simulink model "single_phase_inverter"  (R2020b)
settings: Solver=FixedStepAuto  StartTime=0.0  StopTime=0.3  FixedStep=1e-7  RelTol=1e-3
model workspace (MAT data in the model file):
  ki_u = 1500
  kp_i = 10
  kp_u = 0.1
  m = 0.0001
  n = 1e-06
  time_1 = 0.02
  time_2 = 0.06
undefined symbols (not defined in the file): DiscIntNeverNeededParam
libraries: powerlib x31, pid_lib x6, simulink x2, powerlib_meascontrol x2
settings Model: Creator=csq  LastModifiedBy=csq

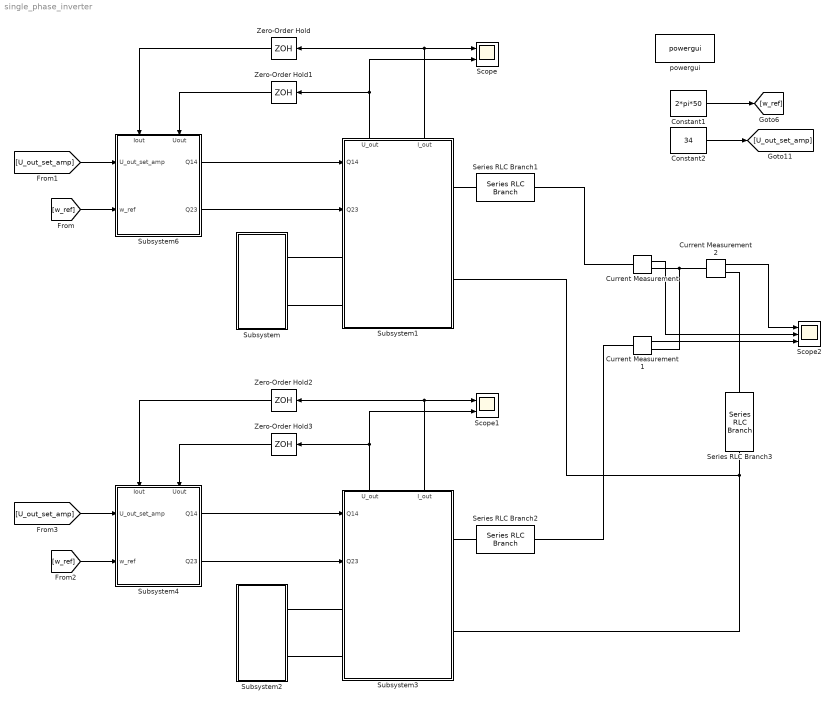
== system single_phase_inverter ==
  Constant1 : Constant  Value=2*pi*50
  Constant2 : Constant  Value=34
  Current Measurement : powerlib/Measurements/Current Measurement  PhasorSimulation=off  OutputType=Complex  PSBequivalent=0
  Current Measurement1 : powerlib/Measurements/Current Measurement  PhasorSimulation=off  OutputType=Complex  PSBequivalent=0
  Current Measurement2 : powerlib/Measurements/Current Measurement  PhasorSimulation=off  OutputType=Complex  PSBequivalent=0
  Scope : Scope  NumInputPorts=2
  Scope1 : Scope  NumInputPorts=2
  Scope2 : Scope  NumInputPorts=3
  Series RLC Branch1 : powerlib/Elements/Series RLC Branch  LConnTagsString=__new0  RConnTagsString=__new0  BranchType=R  Resistance=10e-3  Inductance=1e-3  SetiL0=off  InitialCurrent=0  Capacitance=1e-6  Setx0=off  InitialVoltage=0  Measurements=None
  Series RLC Branch2 : powerlib/Elements/Series RLC Branch  LConnTagsString=__new0  RConnTagsString=__new0  BranchType=R  Resistance=50e-3  Inductance=1e-3  SetiL0=off  InitialCurrent=0  Capacitance=1e-6  Setx0=off  InitialVoltage=0  Measurements=None
  Series RLC Branch3 : powerlib/Elements/Series RLC Branch  LConnTagsString=__new0  RConnTagsString=__new0  BranchType=R  Resistance=12  Inductance=1e-3  SetiL0=off  InitialCurrent=0  Capacitance=1e-6  Setx0=off  InitialVoltage=0  Measurements=None
  Subsystem : Subsystem
  Subsystem1 : Subsystem
      settings: PortSchema="{\"entries\":[{\"content\":{\"sides\":[{\"content\":{\"connectorIds\":[\"In1\",\"In2\",\"LConn1\",\"LConn2\"]},\"type\":\"ConnectorPlacement.EquallySpacedRectSide\",\"uuid\":\"04c4fa80-59b6-45e6-8bac-5e1ed5e22b0f\"},{\"content\":{\"connectorIds\":[\"RConn1\",\"RConn2\"],\"side\":\"RIGHT\"},\"type\":\"ConnectorPlacement.EquallySpacedRectSide\",\"uuid\":\"e41da0a5-fb49-42fc-bfa5-1b3d1422e169\"},{\"content\":{\"connectorIds\":[\"Out1\",\"Out2\"],\"side\":\"TOP\"},\"type\":\"ConnectorPlacement.EquallySpacedRectSide\",\"uuid\":\"69c990dc-7f7f-468a-90c0-dfc1f8754a39\"},{\"content\":{\"connectorIds\":[],\"side\":\"HIDDEN\"},\"type\":\"ConnectorPlacement.EquallySpacedRectSide\",\"uuid\":\"2e87c042-a6fa-4fbf-b837-2a73bea50a04\"}]},\"type\":\"ConnectorPlacement.EquallySpacedConnector\",\"uuid\":\"fc8cbd8d-99a4-408e-86c0-018f445582a3\"}],\"packageUris\":[\"http://schema.mathworks.com/mf0/Connector/R2020b\"],\"version\":\"1.0\"}"
  Subsystem2 : Subsystem
  Subsystem3 : Subsystem
      settings: PortSchema="{\"entries\":[{\"content\":{\"sides\":[{\"content\":{\"connectorIds\":[\"In1\",\"In2\",\"LConn1\",\"LConn2\"]},\"type\":\"ConnectorPlacement.EquallySpacedRectSide\",\"uuid\":\"04c4fa80-59b6-45e6-8bac-5e1ed5e22b0f\"},{\"content\":{\"connectorIds\":[\"RConn1\",\"RConn2\"],\"side\":\"RIGHT\"},\"type\":\"ConnectorPlacement.EquallySpacedRectSide\",\"uuid\":\"e41da0a5-fb49-42fc-bfa5-1b3d1422e169\"},{\"content\":{\"connectorIds\":[\"Out1\",\"Out2\"],\"side\":\"TOP\"},\"type\":\"ConnectorPlacement.EquallySpacedRectSide\",\"uuid\":\"69c990dc-7f7f-468a-90c0-dfc1f8754a39\"},{\"content\":{\"connectorIds\":[],\"side\":\"HIDDEN\"},\"type\":\"ConnectorPlacement.EquallySpacedRectSide\",\"uuid\":\"2e87c042-a6fa-4fbf-b837-2a73bea50a04\"}]},\"type\":\"ConnectorPlacement.EquallySpacedConnector\",\"uuid\":\"fc8cbd8d-99a4-408e-86c0-018f445582a3\"}],\"packageUris\":[\"http://schema.mathworks.com/mf0/Connector/R2020b\"],\"version\":\"1.0\"}"
  Subsystem4 : Subsystem
      settings: PortSchema="{\"entries\":[{\"content\":{\"sides\":[{\"content\":{\"connectorIds\":[\"In1\",\"In2\"]},\"type\":\"ConnectorPlacement.EquallySpacedRectSide\",\"uuid\":\"624b767b-a834-4e37-aaa6-33de15262b98\"},{\"content\":{\"connectorIds\":[\"Out1\",\"Out2\"],\"side\":\"RIGHT\"},\"type\":\"ConnectorPlacement.EquallySpacedRectSide\",\"uuid\":\"636cd8d4-39b1-4a76-b8fe-b877b788af90\"},{\"content\":{\"connectorIds\":[\"In3\",\"In4\"],\"side\":\"TOP\"},\"type\":\"ConnectorPlacement.EquallySpacedRectSide\",\"uuid\":\"27128ec8-804f-46a4-a20c-7bc453791419\"},{\"content\":{\"connectorIds\":[],\"side\":\"HIDDEN\"},\"type\":\"ConnectorPlacement.EquallySpacedRectSide\",\"uuid\":\"cec971ba-b3f6-4dcf-9360-3ebb47930643\"}]},\"type\":\"ConnectorPlacement.EquallySpacedConnector\",\"uuid\":\"76619d1a-6bef-4a4f-ace2-d43c42a45d1f\"}],\"packageUris\":[\"http://schema.mathworks.com/mf0/Connector/R2020b\"],\"version\":\"1.0\"}"
  Subsystem6 : Subsystem
      settings: PortSchema="{\"entries\":[{\"content\":{\"sides\":[{\"content\":{\"connectorIds\":[\"In1\",\"In2\"]},\"type\":\"ConnectorPlacement.EquallySpacedRectSide\",\"uuid\":\"624b767b-a834-4e37-aaa6-33de15262b98\"},{\"content\":{\"connectorIds\":[\"Out1\",\"Out2\"],\"side\":\"RIGHT\"},\"type\":\"ConnectorPlacement.EquallySpacedRectSide\",\"uuid\":\"636cd8d4-39b1-4a76-b8fe-b877b788af90\"},{\"content\":{\"connectorIds\":[\"In3\",\"In4\"],\"side\":\"TOP\"},\"type\":\"ConnectorPlacement.EquallySpacedRectSide\",\"uuid\":\"27128ec8-804f-46a4-a20c-7bc453791419\"},{\"content\":{\"connectorIds\":[],\"side\":\"HIDDEN\"},\"type\":\"ConnectorPlacement.EquallySpacedRectSide\",\"uuid\":\"cec971ba-b3f6-4dcf-9360-3ebb47930643\"}]},\"type\":\"ConnectorPlacement.EquallySpacedConnector\",\"uuid\":\"76619d1a-6bef-4a4f-ace2-d43c42a45d1f\"}],\"packageUris\":[\"http://schema.mathworks.com/mf0/Connector/R2020b\"],\"version\":\"1.0\"}"
  Zero-Order Hold{,1..3} (4 alike) : ZeroOrderHold  SampleTime=1/20e3
  powergui : powerlib/powergui  Priority=1  SimulationMode=Discrete  SampleTime=1e-7  frequency=60  Iterations=50  frequencyindice=0  Pbase=100e6  ErrMax=1e-4  UnitsV=kV  UnitsW=MW  buscounter=0  FunctionMessages=off  echomessages=off  EnableUseOfTLC=off  CurrentSourceSwitches=off  DisableSnubberDevices=off  DisableRonSwitches=off  DisableVfSwitches=off  DisplayEquations=off  AutomaticDiscreteSolvers=off  SolverType=Tustin/Backward Euler (TBE)  Interpol=off  ExternalGateDelay=off  methode=off  Ts=100  x0status=blocks  SPID=on  SwTol=0  HookPort=off  NonlinearTolerance=1e-4  nMaxIteration=100  ContinueOnMaxIteration=off  RestoreLinks=warning  ResistiveCurrentMeasurement=off  Frange=[0:2:500]  Ylog=off  Xlog=on  ShowGrid=off  save=off  variable=ZData  structure=0  ZoomFFT=off  StartTime=0.0  cycles=1  DisplayStyle=1  fundamental=60  FreqAxis=off  MaxFrequency=1000  frequencyindicesteady=1  RmsSteady=1  display=off
  wires:
  Constant1/1 -> [w_ref]
  Constant2/1 -> [U_out_set_amp]
  [w_ref] -> Subsystem6/2(w_ref)
  [U_out_set_amp] -> Subsystem6/1(U_out_set_amp)
  Subsystem6/1(Q14) -> Subsystem1/1(Q14)
  Subsystem6/2(Q23) -> Subsystem1/2(Q23)
  Subsystem1/1(U_out) -> Scope/2, Zero-Order Hold1/1
  Subsystem1/2(I_out) -> Scope/1, Zero-Order Hold/1
  Zero-Order Hold1/1 -> Subsystem6/4(Uout)
  Zero-Order Hold/1 -> Subsystem6/3(Iout)
  Zero-Order Hold2/1 -> Subsystem4/3(Iout)
  Zero-Order Hold3/1 -> Subsystem4/4(Uout)
  Subsystem3/2(I_out) -> Zero-Order Hold2/1, Scope1/1
  Subsystem3/1(U_out) -> Zero-Order Hold3/1, Scope1/2
  [U_out_set_amp] -> Subsystem4/1(U_out_set_amp)
  [w_ref] -> Subsystem4/2(w_ref)
  Subsystem4/1(Q14) -> Subsystem3/1(Q14)
  Subsystem4/2(Q23) -> Subsystem3/2(Q23)
  Current Measurement2/1 -> Scope2/1
  Current Measurement/1 -> Scope2/2
  Current Measurement1/1 -> Scope2/3
  connections:
  Subsystem/RConn1 -- Subsystem1/LConn1
  Subsystem/RConn2 -- Subsystem1/LConn2
  Subsystem2/RConn2 -- Subsystem3/LConn2
  Subsystem2/RConn1 -- Subsystem3/LConn1
  Subsystem1/RConn2 -- Series RLC Branch3/LConn1 -- Subsystem3/RConn2
  Current Measurement/RConn1 -- Current Measurement1/RConn1 -- Current Measurement2/LConn1
  Series RLC Branch3/RConn1 -- Current Measurement2/RConn1
  Subsystem1/RConn1 -- Series RLC Branch1/RConn1
  Subsystem3/RConn1 -- Series RLC Branch2/RConn1
  Series RLC Branch1/LConn1 -- Current Measurement/LConn1
  Series RLC Branch2/LConn1 -- Current Measurement1/LConn1

== system single_phase_inverter/Subsystem ==
  DC Voltage Source1 : powerlib/Electrical Sources/DC Voltage Source  Amplitude=48  Measurements=None
  Series RLC Branch2 : powerlib/Elements/Series RLC Branch  LConnTagsString=__new0  RConnTagsString=__new0  BranchType=R  Resistance=5e-3  Inductance=1e-3  SetiL0=off  InitialCurrent=0  Capacitance=220e-6  Setx0=off  InitialVoltage=0  Measurements=None
  Series RLC Branch6 : powerlib/Elements/Series RLC Branch  LConnTagsString=__new0  RConnTagsString=__new0  BranchType=RC  Resistance=5e-3  Inductance=1e-3  SetiL0=off  InitialCurrent=0  Capacitance=220e-6  Setx0=off  InitialVoltage=0  Measurements=None
  DC+ : PMIOPort  Side=Right
  DC- : PMIOPort  Port=2  Side=Right
  connections:
  DC Voltage Source1/RConn1 -- Series RLC Branch2/RConn1
  DC Voltage Source1/LConn1 -- Series RLC Branch6/RConn1 -- DC-/RConn1
  Series RLC Branch6/LConn1 -- Series RLC Branch2/LConn1 -- DC+/RConn1

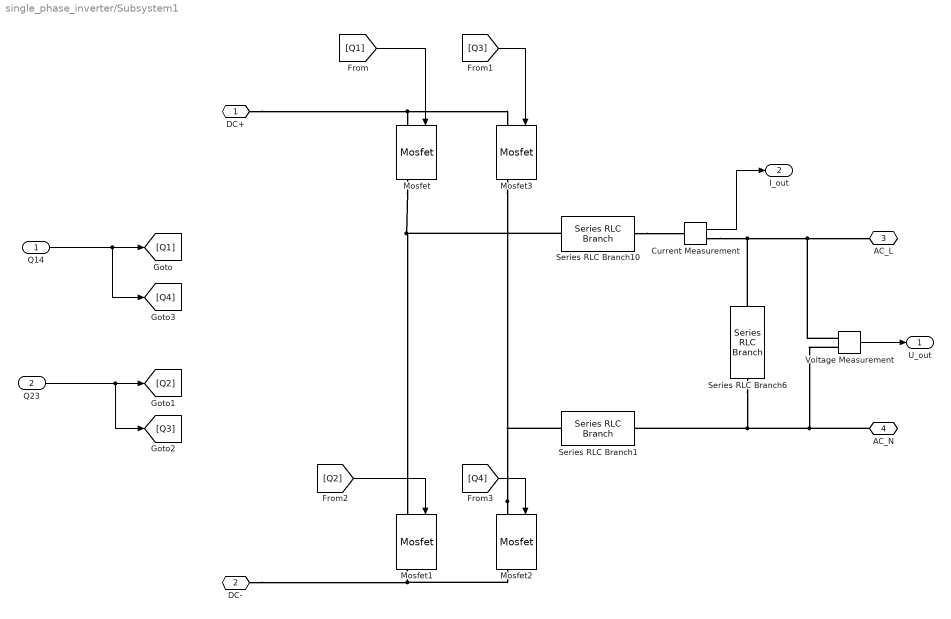
== system single_phase_inverter/Subsystem1 ==
  Q14 : Inport
  Q23 : Inport  Port=2
  Current Measurement : powerlib/Measurements/Current Measurement  PhasorSimulation=off  OutputType=Complex  PSBequivalent=0
  Mosfet{,1..3} (4 alike) : powerlib/Power Electronics/Mosfet  Ron=0.1  Lon=0  Rd=0.01  Vfd=0  IC=0  Rs=1e5  Cs=inf  Measurements=on
  Series RLC Branch1 : powerlib/Elements/Series RLC Branch  LConnTagsString=__new0  RConnTagsString=__new0  BranchType=RL  Resistance=10e-3  Inductance=1e-3  SetiL0=off  InitialCurrent=0  Capacitance=1e-6  Setx0=off  InitialVoltage=0  Measurements=None
  Series RLC Branch10 : powerlib/Elements/Series RLC Branch  LConnTagsString=__new0  RConnTagsString=__new0  BranchType=RL  Resistance=10e-3  Inductance=1e-3  SetiL0=off  InitialCurrent=0  Capacitance=1e-6  Setx0=off  InitialVoltage=0  Measurements=None
  Series RLC Branch6 : powerlib/Elements/Series RLC Branch  LConnTagsString=__new0  RConnTagsString=__new0  BranchType=RC  Resistance=5e-3  Inductance=1e-3  SetiL0=off  InitialCurrent=0  Capacitance=2e-6  Setx0=off  InitialVoltage=0  Measurements=None
  Voltage Measurement : powerlib/Measurements/Voltage Measurement  PhasorSimulation=off  OutputType=Complex  PSBequivalent=0
  DC+ : PMIOPort  Side=Left
  DC- : PMIOPort  Port=2  Side=Left
  AC_L : PMIOPort  Port=3  Side=Right
  AC_N : PMIOPort  Port=4  Side=Right
  U_out : Outport
  I_out : Outport  Port=2
  wires:
  Current Measurement/1 -> I_out/1
  Voltage Measurement/1 -> U_out/1
  [Q1] -> Mosfet/1
  [Q3] -> Mosfet3/1
  [Q2] -> Mosfet1/1
  [Q4] -> Mosfet2/1
  Q23/1 -> [Q3], [Q2]
  Q14/1 -> [Q4], [Q1]
  connections:
  DC-/RConn1 -- Mosfet1/RConn1 -- Mosfet2/RConn1
  DC+/RConn1 -- Mosfet/LConn1 -- Mosfet3/LConn1
  Series RLC Branch6/LConn1 -- Voltage Measurement/LConn1 -- AC_L/RConn1 -- Current Measurement/RConn1
  Mosfet2/LConn1 -- Mosfet3/RConn1 -- Series RLC Branch1/LConn1
  Series RLC Branch10/LConn1 -- Mosfet1/LConn1 -- Mosfet/RConn1
  AC_N/RConn1 -- Series RLC Branch6/RConn1 -- Series RLC Branch1/RConn1 -- Voltage Measurement/LConn2
  Series RLC Branch10/RConn1 -- Current Measurement/LConn1

== system single_phase_inverter/Subsystem2 ==
  DC Voltage Source1 : powerlib/Electrical Sources/DC Voltage Source  Amplitude=48  Measurements=None
  Series RLC Branch2 : powerlib/Elements/Series RLC Branch  LConnTagsString=__new0  RConnTagsString=__new0  BranchType=R  Resistance=5e-3  Inductance=1e-3  SetiL0=off  InitialCurrent=0  Capacitance=220e-6  Setx0=off  InitialVoltage=0  Measurements=None
  Series RLC Branch6 : powerlib/Elements/Series RLC Branch  LConnTagsString=__new0  RConnTagsString=__new0  BranchType=RC  Resistance=5e-3  Inductance=1e-3  SetiL0=off  InitialCurrent=0  Capacitance=220e-6  Setx0=off  InitialVoltage=0  Measurements=None
  DC+ : PMIOPort  Side=Right
  DC- : PMIOPort  Port=2  Side=Right
  connections:
  DC+/RConn1 -- Series RLC Branch6/LConn1 -- Series RLC Branch2/LConn1
  DC-/RConn1 -- Series RLC Branch6/RConn1 -- DC Voltage Source1/LConn1
  DC Voltage Source1/RConn1 -- Series RLC Branch2/RConn1

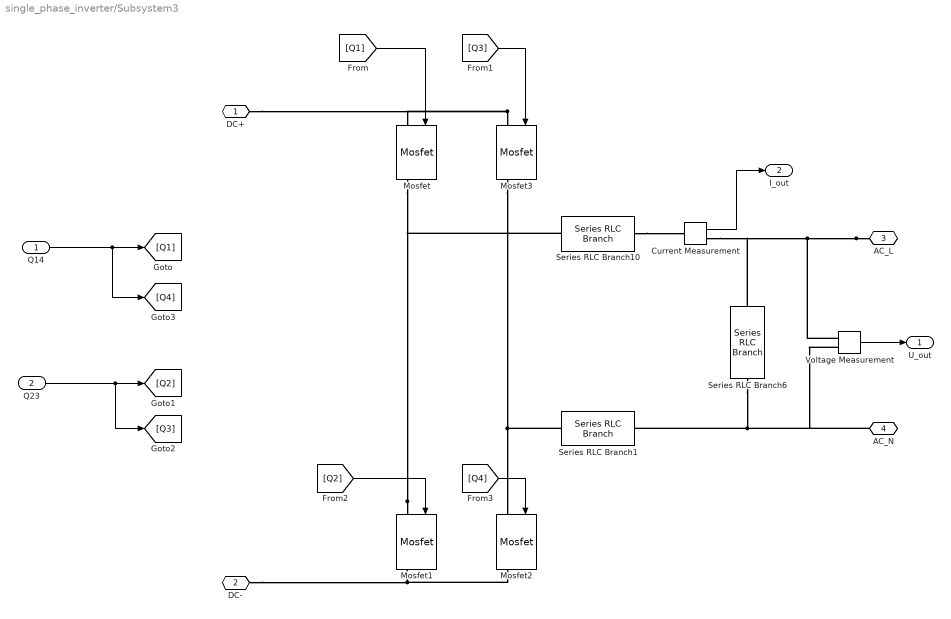
== system single_phase_inverter/Subsystem3 ==
  Q14 : Inport
  Q23 : Inport  Port=2
  Current Measurement : powerlib/Measurements/Current Measurement  PhasorSimulation=off  OutputType=Complex  PSBequivalent=0
  Mosfet{,1..3} (4 alike) : powerlib/Power Electronics/Mosfet  Ron=0.1  Lon=0  Rd=0.01  Vfd=0  IC=0  Rs=1e5  Cs=inf  Measurements=on
  Series RLC Branch1 : powerlib/Elements/Series RLC Branch  LConnTagsString=__new0  RConnTagsString=__new0  BranchType=RL  Resistance=10e-3  Inductance=1e-3  SetiL0=off  InitialCurrent=0  Capacitance=1e-6  Setx0=off  InitialVoltage=0  Measurements=None
  Series RLC Branch10 : powerlib/Elements/Series RLC Branch  LConnTagsString=__new0  RConnTagsString=__new0  BranchType=RL  Resistance=10e-3  Inductance=1e-3  SetiL0=off  InitialCurrent=0  Capacitance=1e-6  Setx0=off  InitialVoltage=0  Measurements=None
  Series RLC Branch6 : powerlib/Elements/Series RLC Branch  LConnTagsString=__new0  RConnTagsString=__new0  BranchType=RC  Resistance=5e-3  Inductance=1e-3  SetiL0=off  InitialCurrent=0  Capacitance=2e-6  Setx0=off  InitialVoltage=0  Measurements=None
  Voltage Measurement : powerlib/Measurements/Voltage Measurement  PhasorSimulation=off  OutputType=Complex  PSBequivalent=0
  DC+ : PMIOPort  Side=Left
  DC- : PMIOPort  Port=2  Side=Left
  AC_L : PMIOPort  Port=3  Side=Right
  AC_N : PMIOPort  Port=4  Side=Right
  U_out : Outport
  I_out : Outport  Port=2
  wires:
  Q14/1 -> [Q1], [Q4]
  Q23/1 -> [Q2], [Q3]
  [Q4] -> Mosfet2/1
  [Q2] -> Mosfet1/1
  [Q3] -> Mosfet3/1
  [Q1] -> Mosfet/1
  Voltage Measurement/1 -> U_out/1
  Current Measurement/1 -> I_out/1
  connections:
  Series RLC Branch10/RConn1 -- Current Measurement/LConn1
  Voltage Measurement/LConn2 -- AC_N/RConn1 -- Series RLC Branch1/RConn1 -- Series RLC Branch6/RConn1
  Mosfet1/LConn1 -- Mosfet/RConn1 -- Series RLC Branch10/LConn1
  Series RLC Branch1/LConn1 -- Mosfet2/LConn1 -- Mosfet3/RConn1
  AC_L/RConn1 -- Voltage Measurement/LConn1 -- Current Measurement/RConn1 -- Series RLC Branch6/LConn1
  Mosfet3/LConn1 -- Mosfet/LConn1 -- DC+/RConn1
  Mosfet2/RConn1 -- Mosfet1/RConn1 -- DC-/RConn1

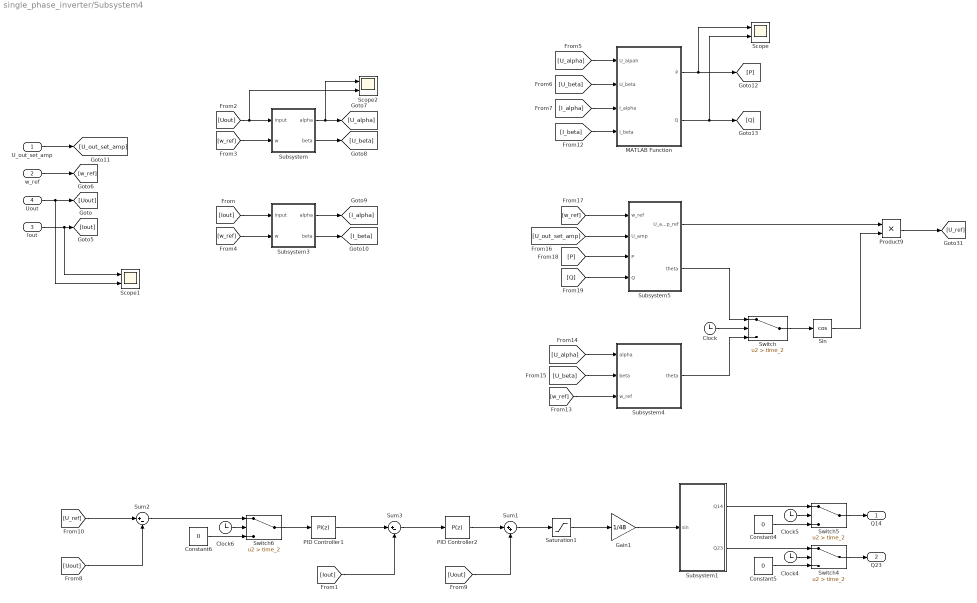
== system single_phase_inverter/Subsystem4 ==
  U_out_set_amp : Inport
  w_ref : Inport  Port=2
  Iout : Inport  Port=3
  Uout : Inport  Port=4
  Clock{,4..6} (4 alike) : Clock
  Constant4 : Constant  Value=0
  Constant5 : Constant  Value=0
  Constant6 : Constant  Value=0
  Gain1 : Gain  Gain=1/48
  MATLAB Function : MATLAB Function  TreatAsAtomicUnit=on
  PID Controller1 : pid_lib/PID Controller  Controller=PI  Form=Parallel  TimeDomain=Discrete-time  UseExternalTs=off  SampleTime=1/20e3  IntegratorMethod=Forward Euler  FilterMethod=Forward Euler  ControllerParametersSource=internal  P=kp_u  I=ki_u  D=0  UseFilter=on  N=100  TunerSelectOption=Transfer Function Based (PID Tuner App)  InitialConditionSource=internal  InitialConditionForIntegrator=0  InitialConditionForFilter=0  DifferentiatorICPrevScaledInput=0  ExternalReset=none  TrackingMode=off  Kt=1  LimitOutput=on  SatLimitsSource=internal  UpperSaturationLimit=50  LowerSaturationLimit=-50  LinearizeAsGain=on  AntiWindupMode=none  Kb=1  POutMin=[]  POutMax=[]  IOutMin=[]  IOutMax=[]  DOutMin=[]  DOutMax=[]  NOutMin=[]  NOutMax=[]  SumOutMin=[]  SumOutMax=[]  SaturationOutMin=[]  SaturationOutMax=[]  PParamMin=[]  PParamMax=[]  IParamMin=[]  IParamMax=[]  DParamMin=[]  DParamMax=[]  NParamMin=[]  NParamMax=[]  KbParamMin=[]  KbParamMax=[]  KtParamMin=[]  KtParamMax=[]  KbOutMin=[]  KbOutMax=[]  KtOutMin=[]  KtOutMax=[]  IntegratorOutMin=[]  IntegratorOutMax=[]  FilterOutMin=[]  FilterOutMax=[]  SumI1OutMin=[]  SumI1OutMax=[]  SumI2OutMin=[]  SumI2OutMax=[]  SumI3OutMin=[]  SumI3OutMax=[]  SumI4OutMin=[]  SumI4OutMax=[]  SumDOutMin=[]  SumDOutMax=[]  DifferentiatorOutMin=[]  DifferentiatorOutMax=[]  FilterDiffOutCoefMin=[]  FilterDiffOutCoefMax=[]  ReciprocalOutMin=[]  ReciprocalOutMax=[]  SumDenOutMin=[]  SumDenOutMax=[]  SumNumOutMin=[]  SumNumOutMax=[]  DivideOutMin=[]  DivideOutMax=[]  UdiffTsProdOutMin=[]  UdiffTsProdOutMax=[]  NTsProdOutMin=[]  NTsProdOutMax=[]  UintegralTsProdOutMin=[]  UintegralTsProdOutMax=[]  UngainTsProdOutMin=[]  UngainTsProdOutMax=[]  IntegratorContinuousStateAttributes=''  IntegratorStateMustResolveToSignalObject=off  IntegratorRTWStateStorageClass=Auto  FilterContinuousStateAttributes=''  FilterStateMustResolveToSignalObject=off  FilterRTWStateStorageClass=Auto  ParallelPVariant=InternalParameters  IdealPVariant=Disabled  IVariant=InternalParameters  DVariant=Disabled  IntegratorVariant=Discrete  SatVariant=Enabled  AWVariant=Passthrough  PCopyVariant=Disabled  TRVariant=Disabled  FdbkBlocksVariant=Forward  IdealPFdbkVariant=Disabled  SatFdbkVariant=Disabled  DerivativeFilterVariant=Disabled  NVariant=Disabled  NCopyVariant=Disabled_SignalSpec  FilterICVariant=Disabled  IntegratorICVariant=InternalICs  ExternalResetVariant=Disabled  TRSumVariant=Passthrough  SumFdbkVariant=Disabled  SumVariant=Sum_PI  TsampFilterVariant=InternalTs  TsampNgainVariant=Passthrough  TsampIntegralVariant=Passthrough  ExternalSaturationOutDataTypeStr=Inherit: Same as second input
  PID Controller2 : pid_lib/PID Controller  Controller=P  Form=Parallel  TimeDomain=Discrete-time  UseExternalTs=off  SampleTime=1/20e3  IntegratorMethod=Forward Euler  FilterMethod=Forward Euler  ControllerParametersSource=internal  P=kp_i  I=10  D=0  UseFilter=on  N=100  TunerSelectOption=Transfer Function Based (PID Tuner App)  InitialConditionSource=internal  InitialConditionForIntegrator=0  InitialConditionForFilter=0  DifferentiatorICPrevScaledInput=0  ExternalReset=none  TrackingMode=off  Kt=1  LimitOutput=off  SatLimitsSource=internal  UpperSaturationLimit=inf  LowerSaturationLimit=-inf  LinearizeAsGain=on  AntiWindupMode=none  Kb=1  POutMin=[]  POutMax=[]  IOutMin=[]  IOutMax=[]  DOutMin=[]  DOutMax=[]  NOutMin=[]  NOutMax=[]  SumOutMin=[]  SumOutMax=[]  SaturationOutMin=[]  SaturationOutMax=[]  PParamMin=[]  PParamMax=[]  IParamMin=[]  IParamMax=[]  DParamMin=[]  DParamMax=[]  NParamMin=[]  NParamMax=[]  KbParamMin=[]  KbParamMax=[]  KtParamMin=[]  KtParamMax=[]  KbOutMin=[]  KbOutMax=[]  KtOutMin=[]  KtOutMax=[]  IntegratorOutMin=[]  IntegratorOutMax=[]  FilterOutMin=[]  FilterOutMax=[]  SumI1OutMin=[]  SumI1OutMax=[]  SumI2OutMin=[]  SumI2OutMax=[]  SumI3OutMin=[]  SumI3OutMax=[]  SumI4OutMin=[]  SumI4OutMax=[]  SumDOutMin=[]  SumDOutMax=[]  DifferentiatorOutMin=[]  DifferentiatorOutMax=[]  FilterDiffOutCoefMin=[]  FilterDiffOutCoefMax=[]  ReciprocalOutMin=[]  ReciprocalOutMax=[]  SumDenOutMin=[]  SumDenOutMax=[]  SumNumOutMin=[]  SumNumOutMax=[]  DivideOutMin=[]  DivideOutMax=[]  UdiffTsProdOutMin=[]  UdiffTsProdOutMax=[]  NTsProdOutMin=[]  NTsProdOutMax=[]  UintegralTsProdOutMin=[]  UintegralTsProdOutMax=[]  UngainTsProdOutMin=[]  UngainTsProdOutMax=[]  IntegratorContinuousStateAttributes=''  IntegratorStateMustResolveToSignalObject=off  IntegratorRTWStateStorageClass=Auto  FilterContinuousStateAttributes=''  FilterStateMustResolveToSignalObject=off  FilterRTWStateStorageClass=Auto  ParallelPVariant=InternalParameters  IdealPVariant=Disabled  IVariant=Disabled  DVariant=Disabled  IntegratorVariant=Disabled  SatVariant=Disabled  AWVariant=Disabled  PCopyVariant=Disabled  TRVariant=Disabled  FdbkBlocksVariant=Forward  IdealPFdbkVariant=Disabled  SatFdbkVariant=Disabled  DerivativeFilterVariant=Disabled  NVariant=Disabled  NCopyVariant=Disabled_SignalSpec  FilterICVariant=Disabled  IntegratorICVariant=Disabled  ExternalResetVariant=Disabled  TRSumVariant=Passthrough  SumFdbkVariant=Disabled  SumVariant=Passthrough_P  TsampFilterVariant=InternalTs  TsampNgainVariant=Passthrough  TsampIntegralVariant=Disabled_SignalSpec  ExternalSaturationOutDataTypeStr=Inherit: Same as second input
  Product9 : Product
  Saturation1 : Saturate  UpperLimit=48  LowerLimit=-48
  Scope : Scope  NumInputPorts=2
  Scope1 : Scope  NumInputPorts=2
  Scope2 : Scope  NumInputPorts=2
  Sin : Trigonometry  Operator=cos
  Subsystem : Subsystem
  Subsystem1 : Subsystem
  Subsystem3 : Subsystem
  Subsystem4 : Subsystem
  Subsystem5 : Subsystem
  Sum1 : Sum  Inputs=|++
  Sum2 : Sum  Inputs=|+-
  Sum3 : Sum  Inputs=|+-
  Switch{,4..6} (4 alike) : Switch  Criteria=u2 > Threshold  Threshold=time_2
  Q14 : Outport
  Q23 : Outport  Port=2
  wires:
  [U_out_set_amp] -> Subsystem5/2(U_amp)
  U_out_set_amp/1 -> [U_out_set_amp]
  w_ref/1 -> [w_ref]
  Uout/1 -> [Uout], Scope1/2
  Iout/1 -> [Iout], Scope1/1
  [U_alpha] -> Subsystem4/1(alpha)
  [U_beta] -> Subsystem4/2(beta)
  Product9/1 -> [U_ref]
  [w_ref] -> Subsystem4/3(w_ref)
  Subsystem3/2(beta) -> [I_beta]
  Subsystem/1(alpha) -> [U_alpha], Scope2/1
  [w_ref] -> Subsystem5/1(w_ref)
  [Q] -> Subsystem5/4(Q)
  [U_alpha] -> MATLAB Function/1(U_alpah)
  Subsystem5/2(theta) -> Switch/1
  Subsystem3/1(alpha) -> [I_alpha]
  [U_beta] -> MATLAB Function/2(U_beta)
  Clock/1 -> Switch/2
  [I_alpha] -> MATLAB Function/3(I_alpha)
  [Iout] -> Subsystem3/1(input)
  [P] -> Subsystem5/3(P)
  [w_ref] -> Subsystem3/2(w)
  Subsystem5/1(U_amp_ref) -> Product9/1
  Subsystem4/1(theta) -> Switch/3
  [Uout] -> Subsystem/1(input), Scope2/2
  Switch/1 -> Sin/1
  Sin/1 -> Product9/2
  Subsystem/2(beta) -> [U_beta]
  MATLAB Function/1(P) -> [P], Scope/1
  MATLAB Function/2(Q) -> [Q], Scope/2
  [I_beta] -> MATLAB Function/4(I_beta)
  [w_ref] -> Subsystem/2(w)
  Constant6/1 -> Switch6/3
  Gain1/1 -> Subsystem1/1(sin)
  Constant4/1 -> Switch5/3
  [Uout] -> Sum1/2
  Switch4/1 -> Q23/1
  Subsystem1/1(Q14) -> Switch5/1
  Switch6/1 -> PID Controller1/1
  Sum2/1 -> Switch6/1
  Subsystem1/2(Q23) -> Switch4/1
  PID Controller2/1 -> Sum1/1
  Clock4/1 -> Switch4/2
  Switch5/1 -> Q14/1
  Constant5/1 -> Switch4/3
  [U_ref] -> Sum2/1
  PID Controller1/1 -> Sum3/1
  Clock6/1 -> Switch6/2
  Saturation1/1 -> Gain1/1
  [Iout] -> Sum3/2
  Clock5/1 -> Switch5/2
  Sum3/1 -> PID Controller2/1
  Sum1/1 -> Saturation1/1
  [Uout] -> Sum2/2

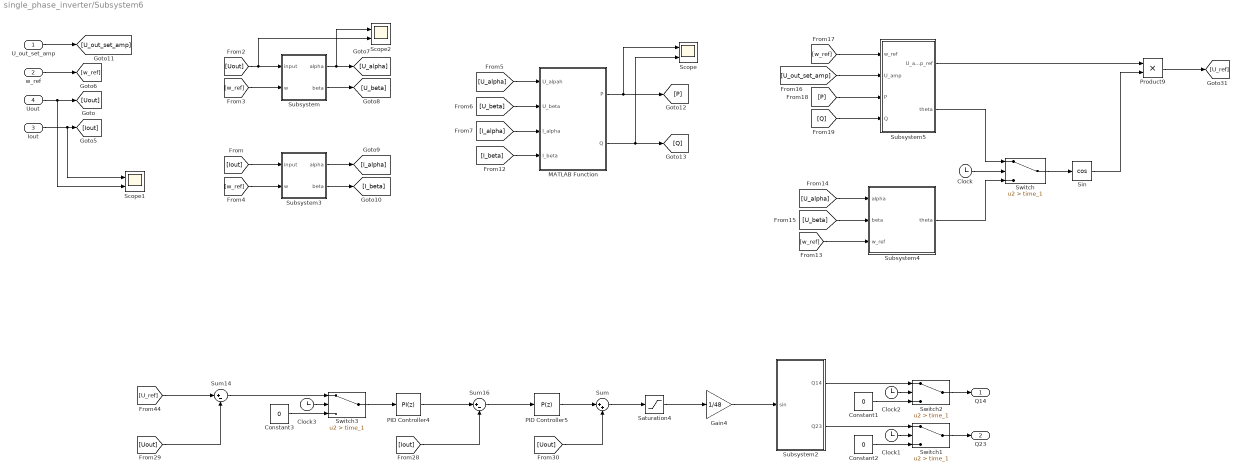
== system single_phase_inverter/Subsystem6 ==
  U_out_set_amp : Inport
  w_ref : Inport  Port=2
  Iout : Inport  Port=3
  Uout : Inport  Port=4
  Clock{,1..3} (4 alike) : Clock
  Constant1 : Constant  Value=0
  Constant2 : Constant  Value=0
  Constant3 : Constant  Value=0
  Gain4 : Gain  Gain=1/48
  MATLAB Function : MATLAB Function  TreatAsAtomicUnit=on
  PID Controller4 : pid_lib/PID Controller  Controller=PI  Form=Parallel  TimeDomain=Discrete-time  UseExternalTs=off  SampleTime=1/20e3  IntegratorMethod=Forward Euler  FilterMethod=Forward Euler  ControllerParametersSource=internal  P=kp_u  I=ki_u  D=0  UseFilter=on  N=100  TunerSelectOption=Transfer Function Based (PID Tuner App)  InitialConditionSource=internal  InitialConditionForIntegrator=0  InitialConditionForFilter=0  DifferentiatorICPrevScaledInput=0  ExternalReset=none  TrackingMode=off  Kt=1  LimitOutput=on  SatLimitsSource=internal  UpperSaturationLimit=50  LowerSaturationLimit=-50  LinearizeAsGain=on  AntiWindupMode=none  Kb=1  POutMin=[]  POutMax=[]  IOutMin=[]  IOutMax=[]  DOutMin=[]  DOutMax=[]  NOutMin=[]  NOutMax=[]  SumOutMin=[]  SumOutMax=[]  SaturationOutMin=[]  SaturationOutMax=[]  PParamMin=[]  PParamMax=[]  IParamMin=[]  IParamMax=[]  DParamMin=[]  DParamMax=[]  NParamMin=[]  NParamMax=[]  KbParamMin=[]  KbParamMax=[]  KtParamMin=[]  KtParamMax=[]  KbOutMin=[]  KbOutMax=[]  KtOutMin=[]  KtOutMax=[]  IntegratorOutMin=[]  IntegratorOutMax=[]  FilterOutMin=[]  FilterOutMax=[]  SumI1OutMin=[]  SumI1OutMax=[]  SumI2OutMin=[]  SumI2OutMax=[]  SumI3OutMin=[]  SumI3OutMax=[]  SumI4OutMin=[]  SumI4OutMax=[]  SumDOutMin=[]  SumDOutMax=[]  DifferentiatorOutMin=[]  DifferentiatorOutMax=[]  FilterDiffOutCoefMin=[]  FilterDiffOutCoefMax=[]  ReciprocalOutMin=[]  ReciprocalOutMax=[]  SumDenOutMin=[]  SumDenOutMax=[]  SumNumOutMin=[]  SumNumOutMax=[]  DivideOutMin=[]  DivideOutMax=[]  UdiffTsProdOutMin=[]  UdiffTsProdOutMax=[]  NTsProdOutMin=[]  NTsProdOutMax=[]  UintegralTsProdOutMin=[]  UintegralTsProdOutMax=[]  UngainTsProdOutMin=[]  UngainTsProdOutMax=[]  IntegratorContinuousStateAttributes=''  IntegratorStateMustResolveToSignalObject=off  IntegratorRTWStateStorageClass=Auto  FilterContinuousStateAttributes=''  FilterStateMustResolveToSignalObject=off  FilterRTWStateStorageClass=Auto  ParallelPVariant=InternalParameters  IdealPVariant=Disabled  IVariant=InternalParameters  DVariant=Disabled  IntegratorVariant=Discrete  SatVariant=Enabled  AWVariant=Passthrough  PCopyVariant=Disabled  TRVariant=Disabled  FdbkBlocksVariant=Forward  IdealPFdbkVariant=Disabled  SatFdbkVariant=Disabled  DerivativeFilterVariant=Disabled  NVariant=Disabled  NCopyVariant=Disabled_SignalSpec  FilterICVariant=Disabled  IntegratorICVariant=InternalICs  ExternalResetVariant=Disabled  TRSumVariant=Passthrough  SumFdbkVariant=Disabled  SumVariant=Sum_PI  TsampFilterVariant=InternalTs  TsampNgainVariant=Passthrough  TsampIntegralVariant=Passthrough  ExternalSaturationOutDataTypeStr=Inherit: Same as second input
  PID Controller5 : pid_lib/PID Controller  Controller=P  Form=Parallel  TimeDomain=Discrete-time  UseExternalTs=off  SampleTime=1/20e3  IntegratorMethod=Forward Euler  FilterMethod=Forward Euler  ControllerParametersSource=internal  P=kp_i  I=10  D=0  UseFilter=on  N=100  TunerSelectOption=Transfer Function Based (PID Tuner App)  InitialConditionSource=internal  InitialConditionForIntegrator=0  InitialConditionForFilter=0  DifferentiatorICPrevScaledInput=0  ExternalReset=none  TrackingMode=off  Kt=1  LimitOutput=off  SatLimitsSource=internal  UpperSaturationLimit=inf  LowerSaturationLimit=-inf  LinearizeAsGain=on  AntiWindupMode=none  Kb=1  POutMin=[]  POutMax=[]  IOutMin=[]  IOutMax=[]  DOutMin=[]  DOutMax=[]  NOutMin=[]  NOutMax=[]  SumOutMin=[]  SumOutMax=[]  SaturationOutMin=[]  SaturationOutMax=[]  PParamMin=[]  PParamMax=[]  IParamMin=[]  IParamMax=[]  DParamMin=[]  DParamMax=[]  NParamMin=[]  NParamMax=[]  KbParamMin=[]  KbParamMax=[]  KtParamMin=[]  KtParamMax=[]  KbOutMin=[]  KbOutMax=[]  KtOutMin=[]  KtOutMax=[]  IntegratorOutMin=[]  IntegratorOutMax=[]  FilterOutMin=[]  FilterOutMax=[]  SumI1OutMin=[]  SumI1OutMax=[]  SumI2OutMin=[]  SumI2OutMax=[]  SumI3OutMin=[]  SumI3OutMax=[]  SumI4OutMin=[]  SumI4OutMax=[]  SumDOutMin=[]  SumDOutMax=[]  DifferentiatorOutMin=[]  DifferentiatorOutMax=[]  FilterDiffOutCoefMin=[]  FilterDiffOutCoefMax=[]  ReciprocalOutMin=[]  ReciprocalOutMax=[]  SumDenOutMin=[]  SumDenOutMax=[]  SumNumOutMin=[]  SumNumOutMax=[]  DivideOutMin=[]  DivideOutMax=[]  UdiffTsProdOutMin=[]  UdiffTsProdOutMax=[]  NTsProdOutMin=[]  NTsProdOutMax=[]  UintegralTsProdOutMin=[]  UintegralTsProdOutMax=[]  UngainTsProdOutMin=[]  UngainTsProdOutMax=[]  IntegratorContinuousStateAttributes=''  IntegratorStateMustResolveToSignalObject=off  IntegratorRTWStateStorageClass=Auto  FilterContinuousStateAttributes=''  FilterStateMustResolveToSignalObject=off  FilterRTWStateStorageClass=Auto  ParallelPVariant=InternalParameters  IdealPVariant=Disabled  IVariant=Disabled  DVariant=Disabled  IntegratorVariant=Disabled  SatVariant=Disabled  AWVariant=Disabled  PCopyVariant=Disabled  TRVariant=Disabled  FdbkBlocksVariant=Forward  IdealPFdbkVariant=Disabled  SatFdbkVariant=Disabled  DerivativeFilterVariant=Disabled  NVariant=Disabled  NCopyVariant=Disabled_SignalSpec  FilterICVariant=Disabled  IntegratorICVariant=Disabled  ExternalResetVariant=Disabled  TRSumVariant=Passthrough  SumFdbkVariant=Disabled  SumVariant=Passthrough_P  TsampFilterVariant=InternalTs  TsampNgainVariant=Passthrough  TsampIntegralVariant=Disabled_SignalSpec  ExternalSaturationOutDataTypeStr=Inherit: Same as second input
  Product9 : Product
  Saturation4 : Saturate  UpperLimit=48  LowerLimit=-48
  Scope : Scope  NumInputPorts=2
  Scope1 : Scope  NumInputPorts=2
  Scope2 : Scope  NumInputPorts=2
  Sin : Trigonometry  Operator=cos
  Subsystem : Subsystem
  Subsystem2 : Subsystem
  Subsystem3 : Subsystem
  Subsystem4 : Subsystem
  Subsystem5 : Subsystem
  Sum : Sum  Inputs=|++
  Sum14 : Sum  Inputs=|+-
  Sum16 : Sum  Inputs=|+-
  Switch{,1..3} (4 alike) : Switch  Criteria=u2 > Threshold  Threshold=time_1
  Q14 : Outport
  Q23 : Outport  Port=2
  wires:
  [w_ref] -> Subsystem/2(w)
  Saturation4/1 -> Gain4/1
  [I_beta] -> MATLAB Function/4(I_beta)
  MATLAB Function/2(Q) -> Scope/2, [Q]
  MATLAB Function/1(P) -> Scope/1, [P]
  Subsystem/2(beta) -> [U_beta]
  Sin/1 -> Product9/2
  Switch/1 -> Sin/1
  [Uout] -> Scope2/2, Subsystem/1(input)
  Subsystem4/1(theta) -> Switch/3
  Subsystem5/1(U_amp_ref) -> Product9/1
  [w_ref] -> Subsystem3/2(w)
  [P] -> Subsystem5/3(P)
  Sum16/1 -> PID Controller5/1
  [Iout] -> Subsystem3/1(input)
  [I_alpha] -> MATLAB Function/3(I_alpha)
  Clock/1 -> Switch/2
  [U_beta] -> MATLAB Function/2(U_beta)
  Subsystem3/1(alpha) -> [I_alpha]
  Subsystem5/2(theta) -> Switch/1
  [U_alpha] -> MATLAB Function/1(U_alpah)
  [Q] -> Subsystem5/4(Q)
  [w_ref] -> Subsystem5/1(w_ref)
  Subsystem/1(alpha) -> Scope2/1, [U_alpha]
  Subsystem3/2(beta) -> [I_beta]
  [w_ref] -> Subsystem4/3(w_ref)
  Product9/1 -> [U_ref]
  [U_beta] -> Subsystem4/2(beta)
  [U_alpha] -> Subsystem4/1(alpha)
  Iout/1 -> Scope1/1, [Iout]
  Uout/1 -> Scope1/2, [Uout]
  w_ref/1 -> [w_ref]
  U_out_set_amp/1 -> [U_out_set_amp]
  Subsystem2/1(Q14) -> Switch2/1
  Constant1/1 -> Switch2/3
  Clock2/1 -> Switch2/2
  Switch2/1 -> Q14/1
  Switch1/1 -> Q23/1
  Clock1/1 -> Switch1/2
  Constant2/1 -> Switch1/3
  Subsystem2/2(Q23) -> Switch1/1
  PID Controller5/1 -> Sum/1
  Sum/1 -> Saturation4/1
  Gain4/1 -> Subsystem2/1(sin)
  Constant3/1 -> Switch3/3
  Clock3/1 -> Switch3/2
  Switch3/1 -> PID Controller4/1
  Sum14/1 -> Switch3/1
  PID Controller4/1 -> Sum16/1
  [U_out_set_amp] -> Subsystem5/2(U_amp)
  [Uout] -> Sum14/2
  [Iout] -> Sum16/2
  [U_ref] -> Sum14/1
  [Uout] -> Sum/2

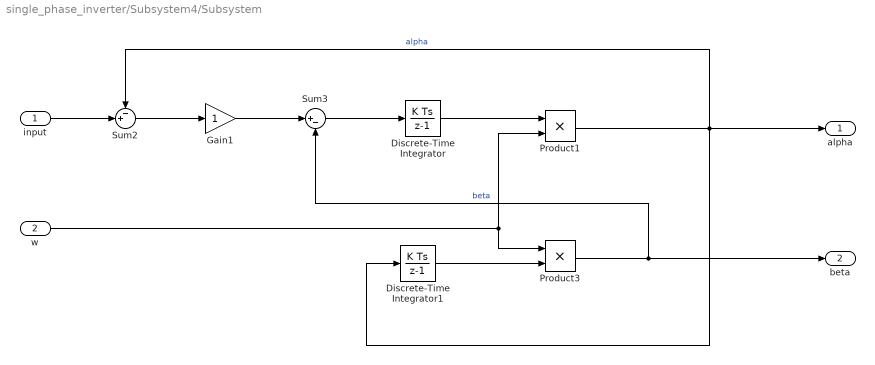
== system single_phase_inverter/Subsystem4/Subsystem ==
  input : Inport
  w : Inport  Port=2
  Discrete-Time Integrator : DiscreteIntegrator  SampleTime=1/20e3  ICPrevOutput=DiscIntNeverNeededParam  ICPrevScaledInput=DiscIntNeverNeededParam
  Discrete-Time Integrator1 : DiscreteIntegrator  SampleTime=1/20e3  ICPrevOutput=DiscIntNeverNeededParam  ICPrevScaledInput=DiscIntNeverNeededParam
  Gain1 : Gain
  Product1 : Product
  Product3 : Product
  Sum2 : Sum  Inputs=-+|
  Sum3 : Sum  Inputs=|+-
  alpha : Outport
  beta : Outport  Port=2
  wires:
  Sum2/1 -> Gain1/1
  Gain1/1 -> Sum3/1
  Product3/1 -> Sum3/2, beta/1  "beta"
  Discrete-Time Integrator/1 -> Product1/1
  Sum3/1 -> Discrete-Time Integrator/1
  Discrete-Time Integrator1/1 -> Product3/2
  input/1 -> Sum2/2
  Product1/1 -> Sum2/1, alpha/1, Discrete-Time Integrator1/1  "alpha"
  w/1 -> Product3/1, Product1/2

== system single_phase_inverter/Subsystem4/Subsystem1 ==
  sin : Inport
  NOT3 : Logic  Operator=NOT  IconShape=distinctive  AllPortsSameDT=off  OutDataTypeStr=boolean
  Relational Operator2 : RelationalOperator  Operator=<  OutDataTypeStr=boolean  RndMeth=Simplest
  Repeating Sequence2 : simulink/Sources/Repeating Sequence  rep_seq_t=[0 1/40e3 1/20e3]  rep_seq_y=[-1 1 -1]
  Q14 : Outport
  Q23 : Outport  Port=2
  wires:
  Repeating Sequence2/1 -> Relational Operator2/1
  NOT3/1 -> Q23/1
  sin/1 -> Relational Operator2/2
  Relational Operator2/1 -> NOT3/1, Q14/1

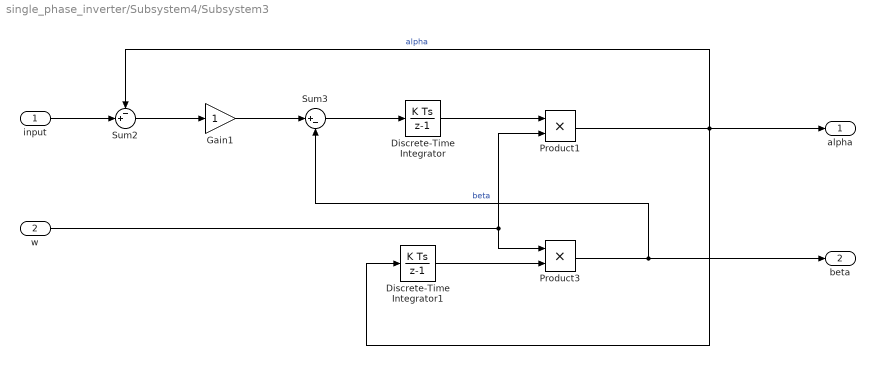
== system single_phase_inverter/Subsystem4/Subsystem3 ==
  input : Inport
  w : Inport  Port=2
  Discrete-Time Integrator : DiscreteIntegrator  SampleTime=1/20e3  ICPrevOutput=DiscIntNeverNeededParam  ICPrevScaledInput=DiscIntNeverNeededParam
  Discrete-Time Integrator1 : DiscreteIntegrator  SampleTime=1/20e3  ICPrevOutput=DiscIntNeverNeededParam  ICPrevScaledInput=DiscIntNeverNeededParam
  Gain1 : Gain
  Product1 : Product
  Product3 : Product
  Sum2 : Sum  Inputs=-+|
  Sum3 : Sum  Inputs=|+-
  alpha : Outport
  beta : Outport  Port=2
  wires:
  w/1 -> Product1/2, Product3/1
  Product1/1 -> Discrete-Time Integrator1/1, alpha/1, Sum2/1  "alpha"
  input/1 -> Sum2/2
  Discrete-Time Integrator1/1 -> Product3/2
  Sum3/1 -> Discrete-Time Integrator/1
  Discrete-Time Integrator/1 -> Product1/1
  Product3/1 -> beta/1, Sum3/2  "beta"
  Gain1/1 -> Sum3/1
  Sum2/1 -> Gain1/1

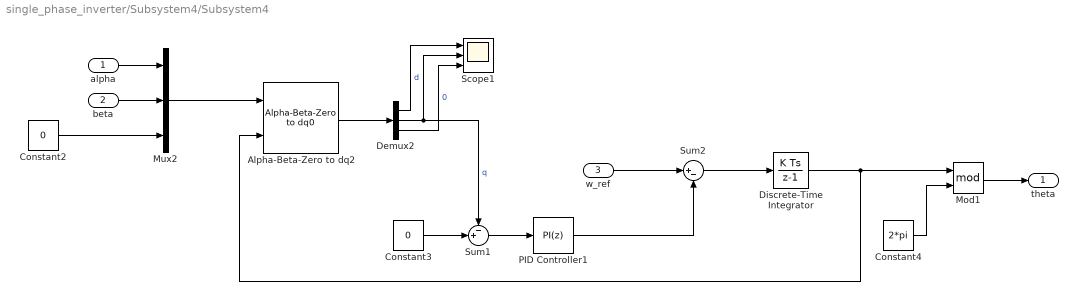
== system single_phase_inverter/Subsystem4/Subsystem4 ==
  alpha : Inport
  beta : Inport  Port=2
  w_ref : Inport  Port=3
  Alpha-Beta-Zero to dq2 : powerlib_meascontrol/Transformations/Alpha-Beta-Zero to dq0  Alignment=Aligned with phase A axis
  Constant2 : Constant  Value=0
  Constant3 : Constant  Value=0
  Constant4 : Constant  Value=2*pi
  Demux2 : Demux  Outputs=3
  Discrete-Time Integrator : DiscreteIntegrator  SampleTime=1/20e3  ICPrevOutput=DiscIntNeverNeededParam  ICPrevScaledInput=DiscIntNeverNeededParam
  Mod1 : Math  Operator=mod  SaturateOnIntegerOverflow=on
  Mux2 : Mux  Inputs=3
  PID Controller1 : pid_lib/PID Controller  Controller=PI  Form=Parallel  TimeDomain=Discrete-time  UseExternalTs=off  SampleTime=1/20e3  IntegratorMethod=Forward Euler  FilterMethod=Forward Euler  ControllerParametersSource=internal  P=0.5  I=0.5  D=0  UseFilter=on  N=100  TunerSelectOption=Transfer Function Based (PID Tuner App)  InitialConditionSource=internal  InitialConditionForIntegrator=0  InitialConditionForFilter=0  DifferentiatorICPrevScaledInput=0  ExternalReset=none  TrackingMode=off  Kt=1  LimitOutput=off  SatLimitsSource=internal  UpperSaturationLimit=inf  LowerSaturationLimit=-inf  LinearizeAsGain=on  AntiWindupMode=none  Kb=1  POutMin=[]  POutMax=[]  IOutMin=[]  IOutMax=[]  DOutMin=[]  DOutMax=[]  NOutMin=[]  NOutMax=[]  SumOutMin=[]  SumOutMax=[]  SaturationOutMin=[]  SaturationOutMax=[]  PParamMin=[]  PParamMax=[]  IParamMin=[]  IParamMax=[]  DParamMin=[]  DParamMax=[]  NParamMin=[]  NParamMax=[]  KbParamMin=[]  KbParamMax=[]  KtParamMin=[]  KtParamMax=[]  KbOutMin=[]  KbOutMax=[]  KtOutMin=[]  KtOutMax=[]  IntegratorOutMin=[]  IntegratorOutMax=[]  FilterOutMin=[]  FilterOutMax=[]  SumI1OutMin=[]  SumI1OutMax=[]  SumI2OutMin=[]  SumI2OutMax=[]  SumI3OutMin=[]  SumI3OutMax=[]  SumI4OutMin=[]  SumI4OutMax=[]  SumDOutMin=[]  SumDOutMax=[]  DifferentiatorOutMin=[]  DifferentiatorOutMax=[]  FilterDiffOutCoefMin=[]  FilterDiffOutCoefMax=[]  ReciprocalOutMin=[]  ReciprocalOutMax=[]  SumDenOutMin=[]  SumDenOutMax=[]  SumNumOutMin=[]  SumNumOutMax=[]  DivideOutMin=[]  DivideOutMax=[]  UdiffTsProdOutMin=[]  UdiffTsProdOutMax=[]  NTsProdOutMin=[]  NTsProdOutMax=[]  UintegralTsProdOutMin=[]  UintegralTsProdOutMax=[]  UngainTsProdOutMin=[]  UngainTsProdOutMax=[]  IntegratorContinuousStateAttributes=''  IntegratorStateMustResolveToSignalObject=off  IntegratorRTWStateStorageClass=Auto  FilterContinuousStateAttributes=''  FilterStateMustResolveToSignalObject=off  FilterRTWStateStorageClass=Auto  ParallelPVariant=InternalParameters  IdealPVariant=Disabled  IVariant=InternalParameters  DVariant=Disabled  IntegratorVariant=Discrete  SatVariant=Disabled  AWVariant=Passthrough  PCopyVariant=Disabled  TRVariant=Disabled  FdbkBlocksVariant=Forward  IdealPFdbkVariant=Disabled  SatFdbkVariant=Disabled  DerivativeFilterVariant=Disabled  NVariant=Disabled  NCopyVariant=Disabled_SignalSpec  FilterICVariant=Disabled  IntegratorICVariant=InternalICs  ExternalResetVariant=Disabled  TRSumVariant=Passthrough  SumFdbkVariant=Disabled  SumVariant=Sum_PI  TsampFilterVariant=InternalTs  TsampNgainVariant=Passthrough  TsampIntegralVariant=Passthrough  ExternalSaturationOutDataTypeStr=Inherit: Same as second input
  Scope1 : Scope  NumInputPorts=3
  Sum1 : Sum  Inputs=-+|
  Sum2 : Sum  Inputs=|+-
  theta : Outport
  wires:
  alpha/1 -> Mux2/1
  Demux2/3 -> Scope1/3  "0"
  PID Controller1/1 -> Sum2/2
  w_ref/1 -> Sum2/1
  Sum2/1 -> Discrete-Time Integrator/1
  Constant3/1 -> Sum1/2
  Constant2/1 -> Mux2/3
  Mod1/1 -> theta/1
  Discrete-Time Integrator/1 -> Alpha-Beta-Zero to dq2/2, Mod1/1
  Constant4/1 -> Mod1/2
  beta/1 -> Mux2/2
  Sum1/1 -> PID Controller1/1
  Demux2/2 -> Sum1/1, Scope1/2  "q"
  Alpha-Beta-Zero to dq2/1 -> Demux2/1
  Mux2/1 -> Alpha-Beta-Zero to dq2/1
  Demux2/1 -> Scope1/1  "d"

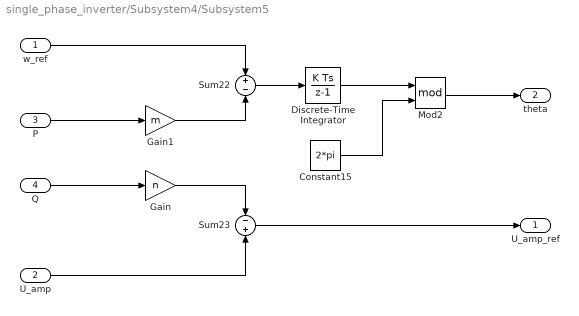
== system single_phase_inverter/Subsystem4/Subsystem5 ==
  w_ref : Inport
  U_amp : Inport  Port=2
  P : Inport  Port=3
  Q : Inport  Port=4
  Constant15 : Constant  Value=2*pi
  Discrete-Time Integrator : DiscreteIntegrator  SampleTime=1/20e3  ICPrevOutput=DiscIntNeverNeededParam  ICPrevScaledInput=DiscIntNeverNeededParam
  Gain : Gain  Gain=n
  Gain1 : Gain  Gain=m
  Mod2 : Math  Operator=mod  SaturateOnIntegerOverflow=on
  Sum22 : Sum  Inputs=+|-
  Sum23 : Sum  Inputs=-|+
  U_amp_ref : Outport
  theta : Outport  Port=2
  wires:
  Q/1 -> Gain/1
  P/1 -> Gain1/1
  w_ref/1 -> Sum22/1
  U_amp/1 -> Sum23/2
  Gain/1 -> Sum23/1
  Sum23/1 -> U_amp_ref/1
  Mod2/1 -> theta/1
  Sum22/1 -> Discrete-Time Integrator/1
  Gain1/1 -> Sum22/2
  Discrete-Time Integrator/1 -> Mod2/1
  Constant15/1 -> Mod2/2

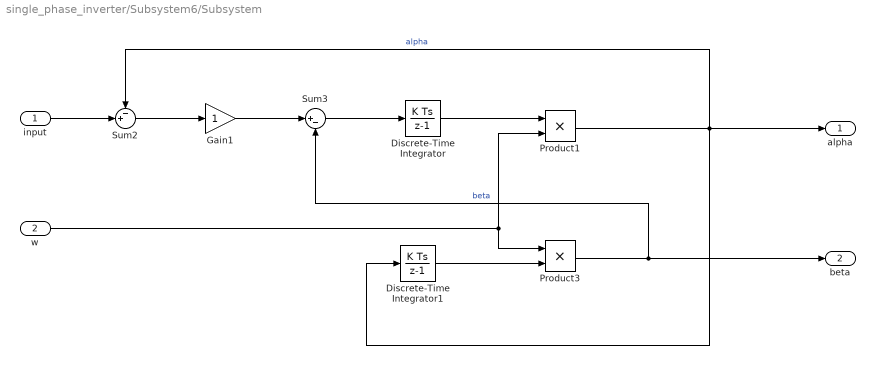
== system single_phase_inverter/Subsystem6/Subsystem ==
  input : Inport
  w : Inport  Port=2
  Discrete-Time Integrator : DiscreteIntegrator  SampleTime=1/20e3  ICPrevOutput=DiscIntNeverNeededParam  ICPrevScaledInput=DiscIntNeverNeededParam
  Discrete-Time Integrator1 : DiscreteIntegrator  SampleTime=1/20e3  ICPrevOutput=DiscIntNeverNeededParam  ICPrevScaledInput=DiscIntNeverNeededParam
  Gain1 : Gain
  Product1 : Product
  Product3 : Product
  Sum2 : Sum  Inputs=-+|
  Sum3 : Sum  Inputs=|+-
  alpha : Outport
  beta : Outport  Port=2
  wires:
  w/1 -> Product1/2, Product3/1
  Product1/1 -> Discrete-Time Integrator1/1, alpha/1, Sum2/1  "alpha"
  input/1 -> Sum2/2
  Discrete-Time Integrator1/1 -> Product3/2
  Sum3/1 -> Discrete-Time Integrator/1
  Discrete-Time Integrator/1 -> Product1/1
  Product3/1 -> beta/1, Sum3/2  "beta"
  Gain1/1 -> Sum3/1
  Sum2/1 -> Gain1/1

== system single_phase_inverter/Subsystem6/Subsystem2 ==
  sin : Inport
  NOT3 : Logic  Operator=NOT  IconShape=distinctive  AllPortsSameDT=off  OutDataTypeStr=boolean
  Relational Operator2 : RelationalOperator  Operator=<  OutDataTypeStr=boolean  RndMeth=Simplest
  Repeating Sequence2 : simulink/Sources/Repeating Sequence  rep_seq_t=[0 1/40e3 1/20e3]  rep_seq_y=[-1 1 -1]
  Q14 : Outport
  Q23 : Outport  Port=2
  wires:
  Repeating Sequence2/1 -> Relational Operator2/1
  NOT3/1 -> Q23/1
  sin/1 -> Relational Operator2/2
  Relational Operator2/1 -> NOT3/1, Q14/1

== system single_phase_inverter/Subsystem6/Subsystem3 ==
  input : Inport
  w : Inport  Port=2
  Discrete-Time Integrator : DiscreteIntegrator  SampleTime=1/20e3  ICPrevOutput=DiscIntNeverNeededParam  ICPrevScaledInput=DiscIntNeverNeededParam
  Discrete-Time Integrator1 : DiscreteIntegrator  SampleTime=1/20e3  ICPrevOutput=DiscIntNeverNeededParam  ICPrevScaledInput=DiscIntNeverNeededParam
  Gain1 : Gain
  Product1 : Product
  Product3 : Product
  Sum2 : Sum  Inputs=-+|
  Sum3 : Sum  Inputs=|+-
  alpha : Outport
  beta : Outport  Port=2
  wires:
  Sum2/1 -> Gain1/1
  Gain1/1 -> Sum3/1
  Product3/1 -> Sum3/2, beta/1  "beta"
  Discrete-Time Integrator/1 -> Product1/1
  Sum3/1 -> Discrete-Time Integrator/1
  Discrete-Time Integrator1/1 -> Product3/2
  input/1 -> Sum2/2
  Product1/1 -> Sum2/1, alpha/1, Discrete-Time Integrator1/1  "alpha"
  w/1 -> Product3/1, Product1/2

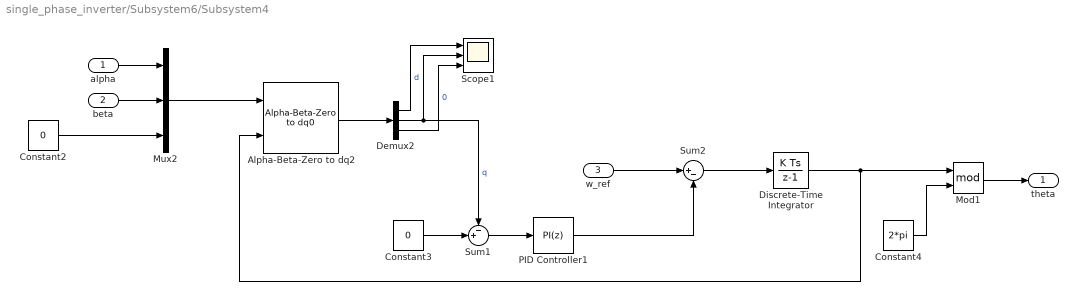
== system single_phase_inverter/Subsystem6/Subsystem4 ==
  alpha : Inport
  beta : Inport  Port=2
  w_ref : Inport  Port=3
  Alpha-Beta-Zero to dq2 : powerlib_meascontrol/Transformations/Alpha-Beta-Zero to dq0  Alignment=Aligned with phase A axis
  Constant2 : Constant  Value=0
  Constant3 : Constant  Value=0
  Constant4 : Constant  Value=2*pi
  Demux2 : Demux  Outputs=3
  Discrete-Time Integrator : DiscreteIntegrator  SampleTime=1/20e3  ICPrevOutput=DiscIntNeverNeededParam  ICPrevScaledInput=DiscIntNeverNeededParam
  Mod1 : Math  Operator=mod  SaturateOnIntegerOverflow=on
  Mux2 : Mux  Inputs=3
  PID Controller1 : pid_lib/PID Controller  Controller=PI  Form=Parallel  TimeDomain=Discrete-time  UseExternalTs=off  SampleTime=1/20e3  IntegratorMethod=Forward Euler  FilterMethod=Forward Euler  ControllerParametersSource=internal  P=0.5  I=0.5  D=0  UseFilter=on  N=100  TunerSelectOption=Transfer Function Based (PID Tuner App)  InitialConditionSource=internal  InitialConditionForIntegrator=0  InitialConditionForFilter=0  DifferentiatorICPrevScaledInput=0  ExternalReset=none  TrackingMode=off  Kt=1  LimitOutput=off  SatLimitsSource=internal  UpperSaturationLimit=inf  LowerSaturationLimit=-inf  LinearizeAsGain=on  AntiWindupMode=none  Kb=1  POutMin=[]  POutMax=[]  IOutMin=[]  IOutMax=[]  DOutMin=[]  DOutMax=[]  NOutMin=[]  NOutMax=[]  SumOutMin=[]  SumOutMax=[]  SaturationOutMin=[]  SaturationOutMax=[]  PParamMin=[]  PParamMax=[]  IParamMin=[]  IParamMax=[]  DParamMin=[]  DParamMax=[]  NParamMin=[]  NParamMax=[]  KbParamMin=[]  KbParamMax=[]  KtParamMin=[]  KtParamMax=[]  KbOutMin=[]  KbOutMax=[]  KtOutMin=[]  KtOutMax=[]  IntegratorOutMin=[]  IntegratorOutMax=[]  FilterOutMin=[]  FilterOutMax=[]  SumI1OutMin=[]  SumI1OutMax=[]  SumI2OutMin=[]  SumI2OutMax=[]  SumI3OutMin=[]  SumI3OutMax=[]  SumI4OutMin=[]  SumI4OutMax=[]  SumDOutMin=[]  SumDOutMax=[]  DifferentiatorOutMin=[]  DifferentiatorOutMax=[]  FilterDiffOutCoefMin=[]  FilterDiffOutCoefMax=[]  ReciprocalOutMin=[]  ReciprocalOutMax=[]  SumDenOutMin=[]  SumDenOutMax=[]  SumNumOutMin=[]  SumNumOutMax=[]  DivideOutMin=[]  DivideOutMax=[]  UdiffTsProdOutMin=[]  UdiffTsProdOutMax=[]  NTsProdOutMin=[]  NTsProdOutMax=[]  UintegralTsProdOutMin=[]  UintegralTsProdOutMax=[]  UngainTsProdOutMin=[]  UngainTsProdOutMax=[]  IntegratorContinuousStateAttributes=''  IntegratorStateMustResolveToSignalObject=off  IntegratorRTWStateStorageClass=Auto  FilterContinuousStateAttributes=''  FilterStateMustResolveToSignalObject=off  FilterRTWStateStorageClass=Auto  ParallelPVariant=InternalParameters  IdealPVariant=Disabled  IVariant=InternalParameters  DVariant=Disabled  IntegratorVariant=Discrete  SatVariant=Disabled  AWVariant=Passthrough  PCopyVariant=Disabled  TRVariant=Disabled  FdbkBlocksVariant=Forward  IdealPFdbkVariant=Disabled  SatFdbkVariant=Disabled  DerivativeFilterVariant=Disabled  NVariant=Disabled  NCopyVariant=Disabled_SignalSpec  FilterICVariant=Disabled  IntegratorICVariant=InternalICs  ExternalResetVariant=Disabled  TRSumVariant=Passthrough  SumFdbkVariant=Disabled  SumVariant=Sum_PI  TsampFilterVariant=InternalTs  TsampNgainVariant=Passthrough  TsampIntegralVariant=Passthrough  ExternalSaturationOutDataTypeStr=Inherit: Same as second input
  Scope1 : Scope  NumInputPorts=3
  Sum1 : Sum  Inputs=-+|
  Sum2 : Sum  Inputs=|+-
  theta : Outport
  wires:
  Demux2/1 -> Scope1/1  "d"
  Mux2/1 -> Alpha-Beta-Zero to dq2/1
  Alpha-Beta-Zero to dq2/1 -> Demux2/1
  Demux2/2 -> Scope1/2, Sum1/1  "q"
  Sum1/1 -> PID Controller1/1
  beta/1 -> Mux2/2
  Constant4/1 -> Mod1/2
  Discrete-Time Integrator/1 -> Mod1/1, Alpha-Beta-Zero to dq2/2
  Mod1/1 -> theta/1
  Constant2/1 -> Mux2/3
  Constant3/1 -> Sum1/2
  Sum2/1 -> Discrete-Time Integrator/1
  w_ref/1 -> Sum2/1
  PID Controller1/1 -> Sum2/2
  Demux2/3 -> Scope1/3  "0"
  alpha/1 -> Mux2/1

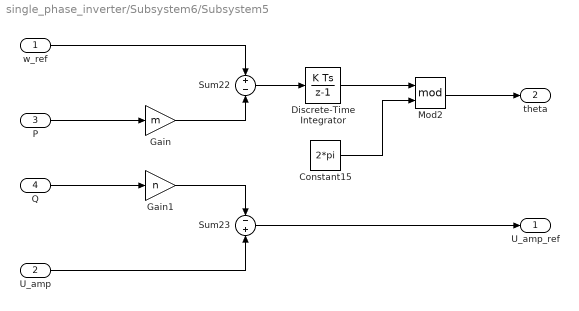
== system single_phase_inverter/Subsystem6/Subsystem5 ==
  w_ref : Inport
  U_amp : Inport  Port=2
  P : Inport  Port=3
  Q : Inport  Port=4
  Constant15 : Constant  Value=2*pi
  Discrete-Time Integrator : DiscreteIntegrator  SampleTime=1/20e3  ICPrevOutput=DiscIntNeverNeededParam  ICPrevScaledInput=DiscIntNeverNeededParam
  Gain : Gain  Gain=m
  Gain1 : Gain  Gain=n
  Mod2 : Math  Operator=mod  SaturateOnIntegerOverflow=on
  Sum22 : Sum  Inputs=+|-
  Sum23 : Sum  Inputs=-|+
  U_amp_ref : Outport
  theta : Outport  Port=2
  wires:
  Constant15/1 -> Mod2/2
  Discrete-Time Integrator/1 -> Mod2/1
  Gain/1 -> Sum22/2
  Sum22/1 -> Discrete-Time Integrator/1
  Mod2/1 -> theta/1
  Sum23/1 -> U_amp_ref/1
  Gain1/1 -> Sum23/1
  U_amp/1 -> Sum23/2
  w_ref/1 -> Sum22/1
  P/1 -> Gain/1
  Q/1 -> Gain1/1

== matlab function single_phase_inverter/Subsystem4/MATLAB Function ==
  data: U_alpah input; P output; U_beta input; I_alpha input; I_beta input; Q output
function [P, Q] = fcn(U_alpah, U_beta, I_alpha, I_beta)

P = (U_alpah * I_alpha + U_beta * I_beta) / 2;
Q = (U_beta * I_alpha - U_alpah * I_beta) / 2;

== matlab function single_phase_inverter/Subsystem6/MATLAB Function ==
  data: U_alpah input; P output; U_beta input; I_alpha input; I_beta input; Q output
function [P, Q] = fcn(U_alpah, U_beta, I_alpha, I_beta)

P = (U_alpah * I_alpha + U_beta * I_beta) / 2;
Q = (U_beta * I_alpha - U_alpah * I_beta) / 2;
